simulink model "ex_2011_11_22_1"  (R2017a)
settings: Solver=FixedStepAuto  StartTime=0.0  StopTime=10.0  FixedStep=0.001  RelTol=1e-3
undefined symbols (not defined in the file or in its folder): aa, b, bet, bet1, d, h, r, T
settings Model: Creator=rastronaut  LastModifiedBy=rastronaut

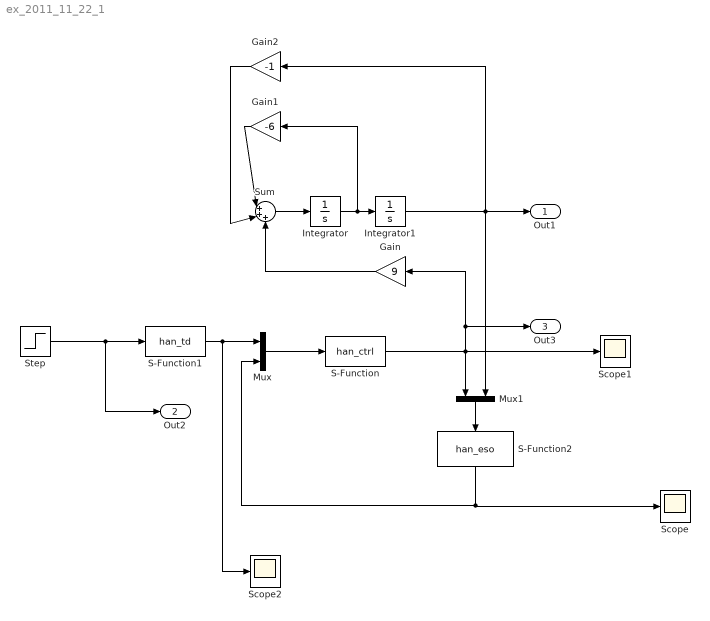
== system ex_2011_11_22_1 ==
  Gain : Gain  Gain=9
  Gain1 : Gain  Gain=-6
  Gain2 : Gain  Gain=-1
  Integrator : Integrator
  Integrator1 : Integrator
  Mux : Mux  Inputs=2
  Mux1 : Mux  Inputs=2
  S-Function : S-Function  FunctionName=han_ctrl  Parameters=aa,bet1,b,d  SFunctionDeploymentMode=off  EnableBusSupport=off
  S-Function1 : S-Function  FunctionName=han_td  Parameters=r,h,T  SFunctionDeploymentMode=off  EnableBusSupport=off
  S-Function2 : S-Function  FunctionName=han_eso  Parameters=d,bet,b,T  SFunctionDeploymentMode=off  EnableBusSupport=off
  Scope : Scope
  Scope1 : Scope
  Scope2 : Scope
  Step : Step  SampleTime=0
  Sum : Sum  Inputs=|+++
  Out1 : Outport  SignalName=Saída
  Out2 : Outport  Port=2  SignalName=Entrada
  Out3 : Outport  Port=3  SignalName=Controle
  wires:
  Mux/1 -> S-Function/1
  Sum/1 -> Integrator/1
  S-Function2/1 -> Scope/1, Mux/2
  S-Function1/1 -> Scope2/1, Mux/1
  Integrator/1 -> Gain1/1, Integrator1/1
  Step/1 -> Out2/1, S-Function1/1
  Mux1/1 -> S-Function2/1
  S-Function/1 -> Scope1/1, Mux1/1, Out3/1, Gain/1
  Integrator1/1 -> Gain2/1, Mux1/2, Out1/1
  Gain/1 -> Sum/3
  Gain1/1 -> Sum/1
  Gain2/1 -> Sum/2
